simulink model "Gain_Scheduler"  (R2019a)
settings: Solver=VariableStepAuto  StartTime=0.0  StopTime=.2  RelTol=1e-3
libraries: sharedschedule x1, cstblocks x1, simulink x1
settings Model: Creator=rag  LastModifiedBy=rag

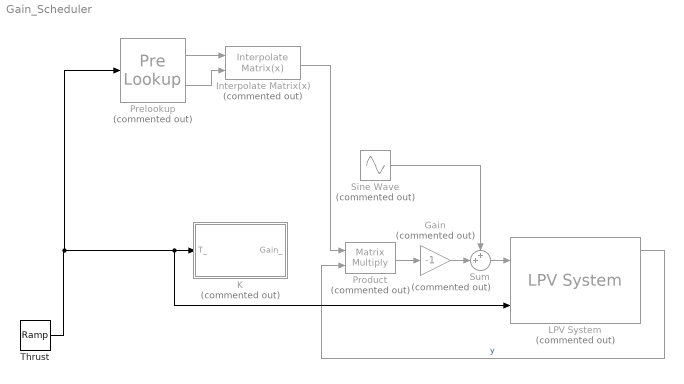
== system Gain_Scheduler ==
  Gain : Gain  Commented=on  Gain=-1
  "Interpolate Matrix(x) " : sharedschedule/Interpolate Matrix(x)   Commented=on  matrix=Krv_Matrix  aMode=aMode
      settings: SourceProductName=Aerospace Blockset  SourceProductBaseCode=AE
  K : MATLAB Function  Commented=on  TreatAsAtomicUnit=on
  LPV System : cstblocks/Linear Parameter Varying/LPV System  Commented=on  sys=ss_sample  x0=0  uOffset=0  yOffset=0  xOffset=0  opEquilOption=on  dxOffset=0  sysFixedOption=Use the first model in state-space array  sysFixed=[]  AFixed=false  BFixed=false  CFixed=false  DFixed=false  uDelayFixed=false  yDelayFixed=false  iDelayFixed=false  IMethod=Linear  EMethod=Clip  IndexSearch=Binary search  IndexBegin=on  OutputX=on  OutputXdot=on  OutputLTI=on  OutputOP=on  DataType=double  SimMode=Interpreted execution  InitBufferSize=1024  FixedBuffer=off
      settings: SourceProductName=Control System Toolbox  SourceProductBaseCode=CT
  Prelookup : PreLookup  Commented=on  BreakpointsData=Thrust_space_lqr  ExtrapMethod=Linear
  Product : Product  Commented=on  Multiplication=Matrix(*)
  Sine Wave : Sin  Commented=on  SampleTime=0
  Sum : Sum  Commented=on  Inputs=++|
  Thrust : simulink/Sources/Ramp  slope=2  start=0  InitialOutput=2
  wires:
  Product/1 -> Gain/1
  LPV System/1 -> Product/2  "y"
  Gain/1 -> Sum/2
  Sum/1 -> LPV System/1
  Thrust/1 -> Prelookup/1, LPV System/2, K/1(T_)
  Prelookup/1 -> "Interpolate Matrix(x) "/1
  Prelookup/2 -> "Interpolate Matrix(x) "/2
  "Interpolate Matrix(x) "/1 -> Product/1
  Sine Wave/1 -> Sum/1

== matlab function Gain_Scheduler/K ==
  data: T_ input; Gain_ output
function Gain_ = fcn(T_)
%#codegen

% Tuned gain surface coefficients
ZERO = zeros(1,1,'like',T_);
Coeffs = cast(reshape([3.21527828158855 0.986873692387624 90.9979817980645 15.7743801117884 0.666789802249185 0.471666013022286 1.45123783040732 0.476508679570159 1.38210308768873 1.37340166641898 -4.46047962467469 -0.388574318445369 -0.350457184974084 -0.705189429322103 0.0186859094502879 26.9539572219363 -0.0134129060378278 0.044674172263538 0.063734170299659 -0.0929941346867395 0.0538223068543678 -0.0786617923883736 -0.0606906216777043 0.137369066641799 0.0251313804703278 -0.136141510331428;-0.24766979201837 2.61243526697287 0.170123401818022 -0.501753482015487 15.8050685299788 0.0274853795270926 0.151783196162779 0.15729080566264 -0.244012925082539 2.21012847770397 -0.0424140262165806 0.079423917427827 -0.15420344817589 -0.211705145650585 -0.664706666257923 -0.155468623770119 0.0240112094031432 0.0517989830542336 0.0253411006118396 0.0159890808770156 -0.147273052202855 0.0555158654823782 -0.356514184019494 -0.184830780942698 0.0417124363567467 0.511425611154544;-0.456646523674522 0.0585314471255562 90.504643497557 0.284030722971712 -0.230613340748825 3.71295602603255 -0.151034758324514 0.548838555019556 0.848003527460162 0.960242082180391 0.25091845243162 0.0755896733104177 4.06402264555677 0.798699024216509 -0.0261649608078235 24.3043855464228 -0.0365627213442141 -0.0693476671432392 -0.110883958491623 0.0374650322362701 -0.0302576765375118 -0.00435493808077856 0.11682368567114 -0.0659205532554247 -0.0186295681366459 -0.264640532492531],[3 13 2]),'like',ZERO);
Offsets = cast(14.5,'like',ZERO);
Scalings = cast(13.5,'like',ZERO);

% Normalization 
T_ = (T_ - Offsets)/Scalings;

% Compute weighted sum of monic terms
deg = 1;
Y = T_;
Gain_ = Coeffs(:,:,1) + Y * Coeffs(:,:,2);
for i=2:deg
   Y = Y * T_;
   Gain_ = Gain_ + Coeffs(:,:,i+1) * Y;
end
